simulink model "contsim"  (Simulink 7.9)
settings: Solver=ode45  StartTime=0.0  StopTime=100  RelTol=1e-3
values from neighbouring files (symbols this model uses):
  A = zeros(5,5,K)    [aaushipcode.m]    (also in contsimu.m = [-betaX 0 0;      0 0 1;      0 0 -betaW]; disc2.m = [-betaX 0 0;      0 0 1;      0 0 -betaW]; discreteship.m = [-5.8/m 0 0;                0 0 1;                0 0 -2]; ncomputation.m = [K K;K*C1 K*C2])
  B = zeros(5,2,K)    [aaushipcode.m]    (also in contsimu.m = [1/m 0;      0 0;      0 1/I]; disc2.m = [1/m 0;      0 0;      0 1/I]; discreteship.m = [0.62/m 0.62/m;                0 0;                0.0305/I ; kalman.m = zeros(9,9,N))
  C = zeros(2,5,K)    [aaushipcode.m]    (also in contsimu.m = [1 0 0;      0 1 0]; disc2.m = [1 0 0;      0 1 0]; discreteship.m = [1 0 0;                0 1 0]; test2.m = [1 0 0;      0 1 0])
  F = zeros(2,5,K)    [aaushipcode.m]    (also in contsimu.m = lqr(A,B,Q,R); disc2.m = lqr(sysD,Q,R); discreteship.m = zeros(2,3,K); ncomputation.m = K*sign(y(1))*y(1)^2 + K*sign(y(2))*y(2)^2)
  N = zeros(2,2,K)    [aaushipcode.m]    (also in contsimu.m = Nuf + F*Nxf; disc2.m = Nuf + F*Nxf; discreteship.m; kalman.m = 5000)
libraries: simulink x1
settings Model: Creator=Lunde  LastModifiedBy=Lunde

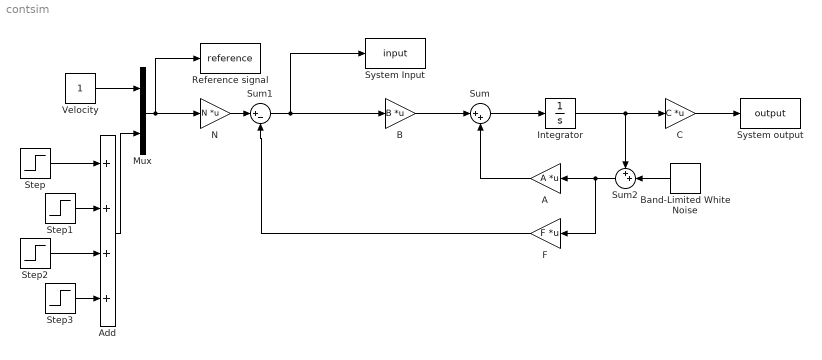
== system contsim ==
  A : Gain  Gain=A  Multiplication=Matrix(K*u)
  Add : Sum  Inputs=++++
  B : Gain  Gain=B  Multiplication=Matrix(K*u)
  Band-Limited White Noise : simulink/Sources/Band-Limited White Noise  Cov=[0.001]  Ts=1  seed=[23341]
  C : Gain  Gain=C  Multiplication=Matrix(K*u)
  F : Gain  Gain=F  Multiplication=Matrix(K*u)
  Integrator : Integrator
  Mux : Mux  Inputs=2
  N : Gain  Gain=N  Multiplication=Matrix(K*u)
  Reference signal : ToWorkspace  VariableName=reference  SampleTime=-1
  Step : Step  Time=0  After=3.14  SampleTime=0
  Step1 : Step  Time=20  After=-3.14  SampleTime=0
  Step2 : Step  Time=40  After=-3.14/2  SampleTime=0
  Step3 : Step  Time=60  After=3.14/2  SampleTime=0
  Sum : Sum  Inputs=|++
  Sum1 : Sum  Inputs=|+-
  Sum2 : Sum  Inputs=++|
  System Input : ToWorkspace  VariableName=input  SampleTime=-1
  System output : ToWorkspace  VariableName=output  SampleTime=-1
  Velocity : Constant
  wires:
  Integrator/1 -> C/1, Sum2/1
  A/1 -> Sum/2
  B/1 -> Sum/1
  Sum/1 -> Integrator/1
  Sum1/1 -> System Input/1, B/1
  F/1 -> Sum1/2
  N/1 -> Sum1/1
  Mux/1 -> N/1, Reference signal/1
  Velocity/1 -> Mux/1
  C/1 -> System output/1
  Sum2/1 -> A/1, F/1
  Band-Limited White Noise/1 -> Sum2/2
  Step1/1 -> Add/2
  Step3/1 -> Add/4
  Step2/1 -> Add/3
  Add/1 -> Mux/2
  Step/1 -> Add/1
